simulink model "question6"  (R2023b)
settings: Solver=VariableStepAuto  StartTime=0.0  StopTime=30  RelTol=1e-3
values from neighbouring files (symbols this model uses):
  A = [-8.8487+(a-b)/5,-0.0399,-5.55+(c+d)/10,3.5846 ... (first row only)    [main_func.m]    (also in question3.m = [-8.8487+(a-b)/5, -0.0399, -5.55+(c+d)/10, 3.5846)
  B = [0.0564+b/(10+c),0.0319 ... (first row only)    [main_func.m]    (also in question3.m = [0.0564+b/(10+c), 0.0319)
  C1 = [1 0 0 0 ... (first row only)    [main_func.m]
  C2 = [0 0 1 0 ... (first row only)    [main_func.m]
  K61 = servo_control_state(A,B,C1,Q1,R1)    [main_func.m]
  K62 = servo_control_state(A,B,C2,Q1,R1)    [main_func.m]
  xsp = [0;0.5;-0.4;0.3]    [main_func.m]
  xsp1 = [0;0.5]    [main_func.m]
  xsp2 = [-0.4;0.3]    [main_func.m]
settings Model: Creator=Fan Xiuqi  LastModifiedBy=Fan Xiuqi

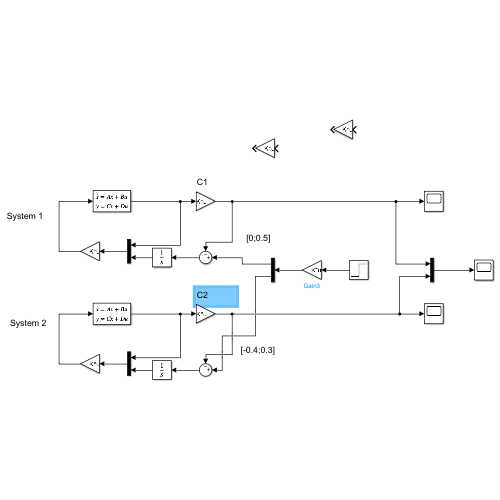
[thumbnail: Simulink's stored preview of the top-level diagram]
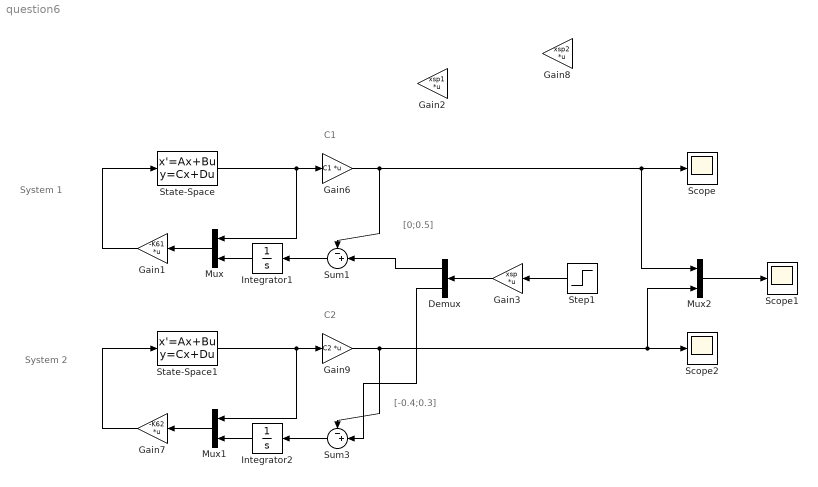
== system question6 ==
  note: System 1
  note: System 2
  note: [0;0.5]
  note: [-0.4;0.3]
  note: C1
  note: C2
  Demux : Demux  Outputs=2
  Gain1 : Gain  Gain=-K61  Multiplication=Matrix(K*u)
  Gain2 : Gain  Gain=xsp1  Multiplication=Matrix(K*u)
  Gain3 : Gain  Gain=xsp  Multiplication=Matrix(K*u)
  Gain6 : Gain  Gain=C1  Multiplication=Matrix(K*u)
  Gain7 : Gain  Gain=-K62  Multiplication=Matrix(K*u)
  Gain8 : Gain  Gain=xsp2  Multiplication=Matrix(K*u)
  Gain9 : Gain  Gain=C2  Multiplication=Matrix(K*u)
  Integrator1 : Integrator
  Integrator2 : Integrator
  Mux : Mux  Inputs=2
  Mux1 : Mux  Inputs=2
  Mux2 : Mux  Inputs=2
  Scope : Scope
  Scope1 : Scope
  Scope2 : Scope
  State-Space : StateSpace  A=A  B=B  C=eye(4)  D=zeros(4,2)  InitialCondition=0
  State-Space1 : StateSpace  A=A  B=B  C=eye(4)  D=zeros(4,2)  InitialCondition=0
  Step1 : Step  SampleTime=0
  Sum1 : Sum  Inputs=-+|
  Sum3 : Sum  Inputs=-+|
  wires:
  Gain1/1 -> State-Space/1
  Step1/1 -> Gain3/1
  State-Space/1 -> Gain6/1, Mux/1
  Integrator1/1 -> Mux/2
  Mux/1 -> Gain1/1
  Sum1/1 -> Integrator1/1
  Gain6/1 -> Sum1/1, Mux2/1, Scope/1
  Gain9/1 -> Mux2/2, Scope2/1, Sum3/1
  Mux1/1 -> Gain7/1
  Integrator2/1 -> Mux1/2
  State-Space1/1 -> Gain9/1, Mux1/1
  Gain7/1 -> State-Space1/1
  Sum3/1 -> Integrator2/1
  Mux2/1 -> Scope1/1
  Gain3/1 -> Demux/1
  Demux/1 -> Sum1/2
  Demux/2 -> Sum3/2
